simulink model "Model"  (R2020b)
settings: Solver=FixedStepDiscrete  StartTime=0.0  StopTime=inf  RelTol=1e-3
undefined symbols (not defined in the file): C12, designMultirateFIR, dt0
libraries: dspmlti4 x96, dspsrcs4 x89
(part 6 of 6)

== system Model/CORE_3_8/Path1/Mixer1 ==
  Input_I : Inport
  Input_Q : Inport  Port=2
  DDS_I : Inport  Port=3
  DDS_Q : Inport  Port=4
  Add : Sum
  Add1 : Sum
  Add2 : Sum  Inputs=-+
  Add3 : Sum  Inputs=+-
  Add4 : Sum
  Delay{1..11} (11 alike) : Delay  DelayLength=1  InitialCondition=0  SampleTime=dt0
  Product : Product
  Product1 : Product
  Product2 : Product
  Output_I : Outport
  Output_Q : Outport  Port=2
  wires:
  DDS_I/1 -> Delay9/1, Add/1
  Input_Q/1 -> Add2/2, Add1/2
  Add/1 -> Delay10/1
  Delay10/1 -> Product/2  "Sum1"
  Add2/1 -> Delay1/1
  Add1/1 -> Delay2/1
  Product/1 -> Delay3/1
  Delay3/1 -> Add4/1, Add3/1  "K1"
  Delay2/1 -> Product1/1  "Sum2"
  Product1/1 -> Delay4/1
  Delay4/1 -> Add3/2  "K2"
  Delay1/1 -> Product2/2  "Sum3"
  Product2/1 -> Delay5/1
  Delay5/1 -> Add4/2  "K3"
  Add3/1 -> Delay6/1
  Add4/1 -> Delay7/1
  Delay6/1 -> Output_I/1  "Sum4"
  Delay7/1 -> Output_Q/1  "Sum5"
  Input_I/1 -> Add2/1, Add1/1, Delay8/1
  DDS_Q/1 -> Delay11/1, Add/2
  Delay8/1 -> Product/1  "Input_I_w1"
  Delay11/1 -> Product1/2  "DDS_Q_w1"
  Delay9/1 -> Product2/1  "DDS_I_w1"

== system Model/CORE_3_8/Path2/DDS_Gen1 ==
  In1 : Inport
  Exp : Math  SaturateOnIntegerOverflow=on
  Gain : Gain  Gain=-1i*2*pi
  Product : Product
  Signal From Workspace1 : dspsrcs4/Signal From Workspace  X=t0  Ts=dt0  nsamps=1  OutputAfterFinalValue=Cyclic repetition  ignoreOrWarnInputAndFrameLengths=off  OutputFrames=off
  Out1 : Outport
  wires:
  Signal From Workspace1/1 -> Gain/1
  Exp/1 -> Out1/1
  Gain/1 -> Product/2
  Product/1 -> Exp/1
  In1/1 -> Product/1

== system Model/CORE_3_8/Path2/Mixer1 ==
  Input_I : Inport
  Input_Q : Inport  Port=2
  DDS_I : Inport  Port=3
  DDS_Q : Inport  Port=4
  Add : Sum
  Add1 : Sum
  Add2 : Sum  Inputs=-+
  Add3 : Sum  Inputs=+-
  Add4 : Sum
  Delay{1..11} (11 alike) : Delay  DelayLength=1  InitialCondition=0  SampleTime=dt0
  Product : Product
  Product1 : Product
  Product2 : Product
  Output_I : Outport
  Output_Q : Outport  Port=2
  wires:
  DDS_I/1 -> Delay9/1, Add/1
  Input_Q/1 -> Add2/2, Add1/2
  Add/1 -> Delay10/1
  Delay10/1 -> Product/2  "Sum1"
  Add2/1 -> Delay1/1
  Add1/1 -> Delay2/1
  Product/1 -> Delay3/1
  Delay3/1 -> Add4/1, Add3/1  "K1"
  Delay2/1 -> Product1/1  "Sum2"
  Product1/1 -> Delay4/1
  Delay4/1 -> Add3/2  "K2"
  Delay1/1 -> Product2/2  "Sum3"
  Product2/1 -> Delay5/1
  Delay5/1 -> Add4/2  "K3"
  Add3/1 -> Delay6/1
  Add4/1 -> Delay7/1
  Delay6/1 -> Output_I/1  "Sum4"
  Delay7/1 -> Output_Q/1  "Sum5"
  Input_I/1 -> Add2/1, Add1/1, Delay8/1
  DDS_Q/1 -> Delay11/1, Add/2
  Delay8/1 -> Product/1  "Input_I_w1"
  Delay11/1 -> Product1/2  "DDS_Q_w1"
  Delay9/1 -> Product2/1  "DDS_I_w1"

== system Model/CORE_3_8/Path3/DDS_Gen1 ==
  In1 : Inport
  Exp : Math  SaturateOnIntegerOverflow=on
  Gain : Gain  Gain=-1i*2*pi
  Product : Product
  Signal From Workspace1 : dspsrcs4/Signal From Workspace  X=t0  Ts=dt0  nsamps=1  OutputAfterFinalValue=Cyclic repetition  ignoreOrWarnInputAndFrameLengths=off  OutputFrames=off
  Out1 : Outport
  wires:
  Signal From Workspace1/1 -> Gain/1
  Exp/1 -> Out1/1
  Gain/1 -> Product/2
  Product/1 -> Exp/1
  In1/1 -> Product/1

== system Model/CORE_3_8/Path3/Mixer1 ==
  Input_I : Inport
  Input_Q : Inport  Port=2
  DDS_I : Inport  Port=3
  DDS_Q : Inport  Port=4
  Add : Sum
  Add1 : Sum
  Add2 : Sum  Inputs=-+
  Add3 : Sum  Inputs=+-
  Add4 : Sum
  Delay{1..11} (11 alike) : Delay  DelayLength=1  InitialCondition=0  SampleTime=dt0
  Product : Product
  Product1 : Product
  Product2 : Product
  Output_I : Outport
  Output_Q : Outport  Port=2
  wires:
  DDS_I/1 -> Delay9/1, Add/1
  Input_Q/1 -> Add2/2, Add1/2
  Add/1 -> Delay10/1
  Delay10/1 -> Product/2  "Sum1"
  Add2/1 -> Delay1/1
  Add1/1 -> Delay2/1
  Product/1 -> Delay3/1
  Delay3/1 -> Add4/1, Add3/1  "K1"
  Delay2/1 -> Product1/1  "Sum2"
  Product1/1 -> Delay4/1
  Delay4/1 -> Add3/2  "K2"
  Delay1/1 -> Product2/2  "Sum3"
  Product2/1 -> Delay5/1
  Delay5/1 -> Add4/2  "K3"
  Add3/1 -> Delay6/1
  Add4/1 -> Delay7/1
  Delay6/1 -> Output_I/1  "Sum4"
  Delay7/1 -> Output_Q/1  "Sum5"
  Input_I/1 -> Add2/1, Add1/1, Delay8/1
  DDS_Q/1 -> Delay11/1, Add/2
  Delay8/1 -> Product/1  "Input_I_w1"
  Delay11/1 -> Product1/2  "DDS_Q_w1"
  Delay9/1 -> Product2/1  "DDS_I_w1"

== system Model/CORE_3_8/Path4/DDS_Gen1 ==
  In1 : Inport
  Exp : Math  SaturateOnIntegerOverflow=on
  Gain : Gain  Gain=-1i*2*pi
  Product : Product
  Signal From Workspace1 : dspsrcs4/Signal From Workspace  X=t0  Ts=dt0  nsamps=1  OutputAfterFinalValue=Cyclic repetition  ignoreOrWarnInputAndFrameLengths=off  OutputFrames=off
  Out1 : Outport
  wires:
  Signal From Workspace1/1 -> Gain/1
  Exp/1 -> Out1/1
  Gain/1 -> Product/2
  Product/1 -> Exp/1
  In1/1 -> Product/1

== system Model/CORE_3_8/Path4/Mixer1 ==
  Input_I : Inport
  Input_Q : Inport  Port=2
  DDS_I : Inport  Port=3
  DDS_Q : Inport  Port=4
  Add : Sum
  Add1 : Sum
  Add2 : Sum  Inputs=-+
  Add3 : Sum  Inputs=+-
  Add4 : Sum
  Delay{1..11} (11 alike) : Delay  DelayLength=1  InitialCondition=0  SampleTime=dt0
  Product : Product
  Product1 : Product
  Product2 : Product
  Output_I : Outport
  Output_Q : Outport  Port=2
  wires:
  DDS_I/1 -> Delay9/1, Add/1
  Input_Q/1 -> Add2/2, Add1/2
  Add/1 -> Delay10/1
  Delay10/1 -> Product/2  "Sum1"
  Add2/1 -> Delay1/1
  Add1/1 -> Delay2/1
  Product/1 -> Delay3/1
  Delay3/1 -> Add4/1, Add3/1  "K1"
  Delay2/1 -> Product1/1  "Sum2"
  Product1/1 -> Delay4/1
  Delay4/1 -> Add3/2  "K2"
  Delay1/1 -> Product2/2  "Sum3"
  Product2/1 -> Delay5/1
  Delay5/1 -> Add4/2  "K3"
  Add3/1 -> Delay6/1
  Add4/1 -> Delay7/1
  Delay6/1 -> Output_I/1  "Sum4"
  Delay7/1 -> Output_Q/1  "Sum5"
  Input_I/1 -> Add2/1, Add1/1, Delay8/1
  DDS_Q/1 -> Delay11/1, Add/2
  Delay8/1 -> Product/1  "Input_I_w1"
  Delay11/1 -> Product1/2  "DDS_Q_w1"
  Delay9/1 -> Product2/1  "DDS_I_w1"

== system Model/CORE_3_8/Path5/DDS_Gen1 ==
  In1 : Inport
  Exp : Math  SaturateOnIntegerOverflow=on
  Gain : Gain  Gain=-1i*2*pi
  Product : Product
  Signal From Workspace1 : dspsrcs4/Signal From Workspace  X=t0  Ts=dt0  nsamps=1  OutputAfterFinalValue=Cyclic repetition  ignoreOrWarnInputAndFrameLengths=off  OutputFrames=off
  Out1 : Outport
  wires:
  Signal From Workspace1/1 -> Gain/1
  Exp/1 -> Out1/1
  Gain/1 -> Product/2
  Product/1 -> Exp/1
  In1/1 -> Product/1

== system Model/CORE_3_8/Path5/Mixer1 ==
  Input_I : Inport
  Input_Q : Inport  Port=2
  DDS_I : Inport  Port=3
  DDS_Q : Inport  Port=4
  Add : Sum
  Add1 : Sum
  Add2 : Sum  Inputs=-+
  Add3 : Sum  Inputs=+-
  Add4 : Sum
  Delay{1..11} (11 alike) : Delay  DelayLength=1  InitialCondition=0  SampleTime=dt0
  Product : Product
  Product1 : Product
  Product2 : Product
  Output_I : Outport
  Output_Q : Outport  Port=2
  wires:
  DDS_I/1 -> Delay9/1, Add/1
  Input_Q/1 -> Add2/2, Add1/2
  Add/1 -> Delay10/1
  Delay10/1 -> Product/2  "Sum1"
  Add2/1 -> Delay1/1
  Add1/1 -> Delay2/1
  Product/1 -> Delay3/1
  Delay3/1 -> Add4/1, Add3/1  "K1"
  Delay2/1 -> Product1/1  "Sum2"
  Product1/1 -> Delay4/1
  Delay4/1 -> Add3/2  "K2"
  Delay1/1 -> Product2/2  "Sum3"
  Product2/1 -> Delay5/1
  Delay5/1 -> Add4/2  "K3"
  Add3/1 -> Delay6/1
  Add4/1 -> Delay7/1
  Delay6/1 -> Output_I/1  "Sum4"
  Delay7/1 -> Output_Q/1  "Sum5"
  Input_I/1 -> Add2/1, Add1/1, Delay8/1
  DDS_Q/1 -> Delay11/1, Add/2
  Delay8/1 -> Product/1  "Input_I_w1"
  Delay11/1 -> Product1/2  "DDS_Q_w1"
  Delay9/1 -> Product2/1  "DDS_I_w1"

== system Model/CORE_3_8/Path6/DDS_Gen1 ==
  In1 : Inport
  Exp : Math  SaturateOnIntegerOverflow=on
  Gain : Gain  Gain=-1i*2*pi
  Product : Product
  Signal From Workspace1 : dspsrcs4/Signal From Workspace  X=t0  Ts=dt0  nsamps=1  OutputAfterFinalValue=Cyclic repetition  ignoreOrWarnInputAndFrameLengths=off  OutputFrames=off
  Out1 : Outport
  wires:
  Signal From Workspace1/1 -> Gain/1
  Exp/1 -> Out1/1
  Gain/1 -> Product/2
  Product/1 -> Exp/1
  In1/1 -> Product/1

== system Model/CORE_3_8/Path6/Mixer1 ==
  Input_I : Inport
  Input_Q : Inport  Port=2
  DDS_I : Inport  Port=3
  DDS_Q : Inport  Port=4
  Add : Sum
  Add1 : Sum
  Add2 : Sum  Inputs=-+
  Add3 : Sum  Inputs=+-
  Add4 : Sum
  Delay{1..11} (11 alike) : Delay  DelayLength=1  InitialCondition=0  SampleTime=dt0
  Product : Product
  Product1 : Product
  Product2 : Product
  Output_I : Outport
  Output_Q : Outport  Port=2
  wires:
  DDS_I/1 -> Delay9/1, Add/1
  Input_Q/1 -> Add2/2, Add1/2
  Add/1 -> Delay10/1
  Delay10/1 -> Product/2  "Sum1"
  Add2/1 -> Delay1/1
  Add1/1 -> Delay2/1
  Product/1 -> Delay3/1
  Delay3/1 -> Add4/1, Add3/1  "K1"
  Delay2/1 -> Product1/1  "Sum2"
  Product1/1 -> Delay4/1
  Delay4/1 -> Add3/2  "K2"
  Delay1/1 -> Product2/2  "Sum3"
  Product2/1 -> Delay5/1
  Delay5/1 -> Add4/2  "K3"
  Add3/1 -> Delay6/1
  Add4/1 -> Delay7/1
  Delay6/1 -> Output_I/1  "Sum4"
  Delay7/1 -> Output_Q/1  "Sum5"
  Input_I/1 -> Add2/1, Add1/1, Delay8/1
  DDS_Q/1 -> Delay11/1, Add/2
  Delay8/1 -> Product/1  "Input_I_w1"
  Delay11/1 -> Product1/2  "DDS_Q_w1"
  Delay9/1 -> Product2/1  "DDS_I_w1"

== system Model/CORE_3_8/Path7/DDS_Gen1 ==
  In1 : Inport
  Exp : Math  SaturateOnIntegerOverflow=on
  Gain : Gain  Gain=-1i*2*pi
  Product : Product
  Signal From Workspace1 : dspsrcs4/Signal From Workspace  X=t0  Ts=dt0  nsamps=1  OutputAfterFinalValue=Cyclic repetition  ignoreOrWarnInputAndFrameLengths=off  OutputFrames=off
  Out1 : Outport
  wires:
  Signal From Workspace1/1 -> Gain/1
  Exp/1 -> Out1/1
  Gain/1 -> Product/2
  Product/1 -> Exp/1
  In1/1 -> Product/1

== system Model/CORE_3_8/Path7/Mixer1 ==
  Input_I : Inport
  Input_Q : Inport  Port=2
  DDS_I : Inport  Port=3
  DDS_Q : Inport  Port=4
  Add : Sum
  Add1 : Sum
  Add2 : Sum  Inputs=-+
  Add3 : Sum  Inputs=+-
  Add4 : Sum
  Delay{1..11} (11 alike) : Delay  DelayLength=1  InitialCondition=0  SampleTime=dt0
  Product : Product
  Product1 : Product
  Product2 : Product
  Output_I : Outport
  Output_Q : Outport  Port=2
  wires:
  DDS_I/1 -> Delay9/1, Add/1
  Input_Q/1 -> Add2/2, Add1/2
  Add/1 -> Delay10/1
  Delay10/1 -> Product/2  "Sum1"
  Add2/1 -> Delay1/1
  Add1/1 -> Delay2/1
  Product/1 -> Delay3/1
  Delay3/1 -> Add4/1, Add3/1  "K1"
  Delay2/1 -> Product1/1  "Sum2"
  Product1/1 -> Delay4/1
  Delay4/1 -> Add3/2  "K2"
  Delay1/1 -> Product2/2  "Sum3"
  Product2/1 -> Delay5/1
  Delay5/1 -> Add4/2  "K3"
  Add3/1 -> Delay6/1
  Add4/1 -> Delay7/1
  Delay6/1 -> Output_I/1  "Sum4"
  Delay7/1 -> Output_Q/1  "Sum5"
  Input_I/1 -> Add2/1, Add1/1, Delay8/1
  DDS_Q/1 -> Delay11/1, Add/2
  Delay8/1 -> Product/1  "Input_I_w1"
  Delay11/1 -> Product1/2  "DDS_Q_w1"
  Delay9/1 -> Product2/1  "DDS_I_w1"

== system Model/CORE_3_8/Path8/DDS_Gen1 ==
  In1 : Inport
  Exp : Math  SaturateOnIntegerOverflow=on
  Gain : Gain  Gain=-1i*2*pi
  Product : Product
  Signal From Workspace1 : dspsrcs4/Signal From Workspace  X=t0  Ts=dt0  nsamps=1  OutputAfterFinalValue=Cyclic repetition  ignoreOrWarnInputAndFrameLengths=off  OutputFrames=off
  Out1 : Outport
  wires:
  Signal From Workspace1/1 -> Gain/1
  Exp/1 -> Out1/1
  Gain/1 -> Product/2
  Product/1 -> Exp/1
  In1/1 -> Product/1

== system Model/CORE_3_8/Path8/Mixer1 ==
  Input_I : Inport
  Input_Q : Inport  Port=2
  DDS_I : Inport  Port=3
  DDS_Q : Inport  Port=4
  Add : Sum
  Add1 : Sum
  Add2 : Sum  Inputs=-+
  Add3 : Sum  Inputs=+-
  Add4 : Sum
  Delay{1..11} (11 alike) : Delay  DelayLength=1  InitialCondition=0  SampleTime=dt0
  Product : Product
  Product1 : Product
  Product2 : Product
  Output_I : Outport
  Output_Q : Outport  Port=2
  wires:
  DDS_I/1 -> Delay9/1, Add/1
  Input_Q/1 -> Add2/2, Add1/2
  Add/1 -> Delay10/1
  Delay10/1 -> Product/2  "Sum1"
  Add2/1 -> Delay1/1
  Add1/1 -> Delay2/1
  Product/1 -> Delay3/1
  Delay3/1 -> Add4/1, Add3/1  "K1"
  Delay2/1 -> Product1/1  "Sum2"
  Product1/1 -> Delay4/1
  Delay4/1 -> Add3/2  "K2"
  Delay1/1 -> Product2/2  "Sum3"
  Product2/1 -> Delay5/1
  Delay5/1 -> Add4/2  "K3"
  Add3/1 -> Delay6/1
  Add4/1 -> Delay7/1
  Delay6/1 -> Output_I/1  "Sum4"
  Delay7/1 -> Output_Q/1  "Sum5"
  Input_I/1 -> Add2/1, Add1/1, Delay8/1
  DDS_Q/1 -> Delay11/1, Add/2
  Delay8/1 -> Product/1  "Input_I_w1"
  Delay11/1 -> Product1/2  "DDS_Q_w1"
  Delay9/1 -> Product2/1  "DDS_I_w1"

== system Model/CORE_3_9/Path1/DDS_Gen1 ==
  In1 : Inport
  Exp : Math  SaturateOnIntegerOverflow=on
  Gain : Gain  Gain=-1i*2*pi
  Product : Product
  Signal From Workspace1 : dspsrcs4/Signal From Workspace  X=t0  Ts=dt0  nsamps=1  OutputAfterFinalValue=Cyclic repetition  ignoreOrWarnInputAndFrameLengths=off  OutputFrames=off
  Out1 : Outport
  wires:
  Signal From Workspace1/1 -> Gain/1
  Exp/1 -> Out1/1
  Gain/1 -> Product/2
  Product/1 -> Exp/1
  In1/1 -> Product/1

== system Model/CORE_3_9/Path1/Mixer1 ==
  Input_I : Inport
  Input_Q : Inport  Port=2
  DDS_I : Inport  Port=3
  DDS_Q : Inport  Port=4
  Add : Sum
  Add1 : Sum
  Add2 : Sum  Inputs=-+
  Add3 : Sum  Inputs=+-
  Add4 : Sum
  Delay{1..11} (11 alike) : Delay  DelayLength=1  InitialCondition=0  SampleTime=dt0
  Product : Product
  Product1 : Product
  Product2 : Product
  Output_I : Outport
  Output_Q : Outport  Port=2
  wires:
  DDS_I/1 -> Delay9/1, Add/1
  Input_Q/1 -> Add2/2, Add1/2
  Add/1 -> Delay10/1
  Delay10/1 -> Product/2  "Sum1"
  Add2/1 -> Delay1/1
  Add1/1 -> Delay2/1
  Product/1 -> Delay3/1
  Delay3/1 -> Add4/1, Add3/1  "K1"
  Delay2/1 -> Product1/1  "Sum2"
  Product1/1 -> Delay4/1
  Delay4/1 -> Add3/2  "K2"
  Delay1/1 -> Product2/2  "Sum3"
  Product2/1 -> Delay5/1
  Delay5/1 -> Add4/2  "K3"
  Add3/1 -> Delay6/1
  Add4/1 -> Delay7/1
  Delay6/1 -> Output_I/1  "Sum4"
  Delay7/1 -> Output_Q/1  "Sum5"
  Input_I/1 -> Add2/1, Add1/1, Delay8/1
  DDS_Q/1 -> Delay11/1, Add/2
  Delay8/1 -> Product/1  "Input_I_w1"
  Delay11/1 -> Product1/2  "DDS_Q_w1"
  Delay9/1 -> Product2/1  "DDS_I_w1"

== system Model/CORE_3_9/Path2/DDS_Gen1 ==
  In1 : Inport
  Exp : Math  SaturateOnIntegerOverflow=on
  Gain : Gain  Gain=-1i*2*pi
  Product : Product
  Signal From Workspace1 : dspsrcs4/Signal From Workspace  X=t0  Ts=dt0  nsamps=1  OutputAfterFinalValue=Cyclic repetition  ignoreOrWarnInputAndFrameLengths=off  OutputFrames=off
  Out1 : Outport
  wires:
  Signal From Workspace1/1 -> Gain/1
  Exp/1 -> Out1/1
  Gain/1 -> Product/2
  Product/1 -> Exp/1
  In1/1 -> Product/1

== system Model/CORE_3_9/Path2/Mixer1 ==
  Input_I : Inport
  Input_Q : Inport  Port=2
  DDS_I : Inport  Port=3
  DDS_Q : Inport  Port=4
  Add : Sum
  Add1 : Sum
  Add2 : Sum  Inputs=-+
  Add3 : Sum  Inputs=+-
  Add4 : Sum
  Delay{1..11} (11 alike) : Delay  DelayLength=1  InitialCondition=0  SampleTime=dt0
  Product : Product
  Product1 : Product
  Product2 : Product
  Output_I : Outport
  Output_Q : Outport  Port=2
  wires:
  DDS_I/1 -> Delay9/1, Add/1
  Input_Q/1 -> Add2/2, Add1/2
  Add/1 -> Delay10/1
  Delay10/1 -> Product/2  "Sum1"
  Add2/1 -> Delay1/1
  Add1/1 -> Delay2/1
  Product/1 -> Delay3/1
  Delay3/1 -> Add4/1, Add3/1  "K1"
  Delay2/1 -> Product1/1  "Sum2"
  Product1/1 -> Delay4/1
  Delay4/1 -> Add3/2  "K2"
  Delay1/1 -> Product2/2  "Sum3"
  Product2/1 -> Delay5/1
  Delay5/1 -> Add4/2  "K3"
  Add3/1 -> Delay6/1
  Add4/1 -> Delay7/1
  Delay6/1 -> Output_I/1  "Sum4"
  Delay7/1 -> Output_Q/1  "Sum5"
  Input_I/1 -> Add2/1, Add1/1, Delay8/1
  DDS_Q/1 -> Delay11/1, Add/2
  Delay8/1 -> Product/1  "Input_I_w1"
  Delay11/1 -> Product1/2  "DDS_Q_w1"
  Delay9/1 -> Product2/1  "DDS_I_w1"

== system Model/CORE_3_9/Path3/DDS_Gen1 ==
  In1 : Inport
  Exp : Math  SaturateOnIntegerOverflow=on
  Gain : Gain  Gain=-1i*2*pi
  Product : Product
  Signal From Workspace1 : dspsrcs4/Signal From Workspace  X=t0  Ts=dt0  nsamps=1  OutputAfterFinalValue=Cyclic repetition  ignoreOrWarnInputAndFrameLengths=off  OutputFrames=off
  Out1 : Outport
  wires:
  Signal From Workspace1/1 -> Gain/1
  Exp/1 -> Out1/1
  Gain/1 -> Product/2
  Product/1 -> Exp/1
  In1/1 -> Product/1

== system Model/CORE_3_9/Path3/Mixer1 ==
  Input_I : Inport
  Input_Q : Inport  Port=2
  DDS_I : Inport  Port=3
  DDS_Q : Inport  Port=4
  Add : Sum
  Add1 : Sum
  Add2 : Sum  Inputs=-+
  Add3 : Sum  Inputs=+-
  Add4 : Sum
  Delay{1..11} (11 alike) : Delay  DelayLength=1  InitialCondition=0  SampleTime=dt0
  Product : Product
  Product1 : Product
  Product2 : Product
  Output_I : Outport
  Output_Q : Outport  Port=2
  wires:
  DDS_I/1 -> Delay9/1, Add/1
  Input_Q/1 -> Add2/2, Add1/2
  Add/1 -> Delay10/1
  Delay10/1 -> Product/2  "Sum1"
  Add2/1 -> Delay1/1
  Add1/1 -> Delay2/1
  Product/1 -> Delay3/1
  Delay3/1 -> Add4/1, Add3/1  "K1"
  Delay2/1 -> Product1/1  "Sum2"
  Product1/1 -> Delay4/1
  Delay4/1 -> Add3/2  "K2"
  Delay1/1 -> Product2/2  "Sum3"
  Product2/1 -> Delay5/1
  Delay5/1 -> Add4/2  "K3"
  Add3/1 -> Delay6/1
  Add4/1 -> Delay7/1
  Delay6/1 -> Output_I/1  "Sum4"
  Delay7/1 -> Output_Q/1  "Sum5"
  Input_I/1 -> Add2/1, Add1/1, Delay8/1
  DDS_Q/1 -> Delay11/1, Add/2
  Delay8/1 -> Product/1  "Input_I_w1"
  Delay11/1 -> Product1/2  "DDS_Q_w1"
  Delay9/1 -> Product2/1  "DDS_I_w1"

== system Model/CORE_3_9/Path4/DDS_Gen1 ==
  In1 : Inport
  Exp : Math  SaturateOnIntegerOverflow=on
  Gain : Gain  Gain=-1i*2*pi
  Product : Product
  Signal From Workspace1 : dspsrcs4/Signal From Workspace  X=t0  Ts=dt0  nsamps=1  OutputAfterFinalValue=Cyclic repetition  ignoreOrWarnInputAndFrameLengths=off  OutputFrames=off
  Out1 : Outport
  wires:
  Signal From Workspace1/1 -> Gain/1
  Exp/1 -> Out1/1
  Gain/1 -> Product/2
  Product/1 -> Exp/1
  In1/1 -> Product/1

== system Model/CORE_3_9/Path4/Mixer1 ==
  Input_I : Inport
  Input_Q : Inport  Port=2
  DDS_I : Inport  Port=3
  DDS_Q : Inport  Port=4
  Add : Sum
  Add1 : Sum
  Add2 : Sum  Inputs=-+
  Add3 : Sum  Inputs=+-
  Add4 : Sum
  Delay{1..11} (11 alike) : Delay  DelayLength=1  InitialCondition=0  SampleTime=dt0
  Product : Product
  Product1 : Product
  Product2 : Product
  Output_I : Outport
  Output_Q : Outport  Port=2
  wires:
  DDS_I/1 -> Delay9/1, Add/1
  Input_Q/1 -> Add2/2, Add1/2
  Add/1 -> Delay10/1
  Delay10/1 -> Product/2  "Sum1"
  Add2/1 -> Delay1/1
  Add1/1 -> Delay2/1
  Product/1 -> Delay3/1
  Delay3/1 -> Add4/1, Add3/1  "K1"
  Delay2/1 -> Product1/1  "Sum2"
  Product1/1 -> Delay4/1
  Delay4/1 -> Add3/2  "K2"
  Delay1/1 -> Product2/2  "Sum3"
  Product2/1 -> Delay5/1
  Delay5/1 -> Add4/2  "K3"
  Add3/1 -> Delay6/1
  Add4/1 -> Delay7/1
  Delay6/1 -> Output_I/1  "Sum4"
  Delay7/1 -> Output_Q/1  "Sum5"
  Input_I/1 -> Add2/1, Add1/1, Delay8/1
  DDS_Q/1 -> Delay11/1, Add/2
  Delay8/1 -> Product/1  "Input_I_w1"
  Delay11/1 -> Product1/2  "DDS_Q_w1"
  Delay9/1 -> Product2/1  "DDS_I_w1"

== system Model/CORE_3_9/Path5/DDS_Gen1 ==
  In1 : Inport
  Exp : Math  SaturateOnIntegerOverflow=on
  Gain : Gain  Gain=-1i*2*pi
  Product : Product
  Signal From Workspace1 : dspsrcs4/Signal From Workspace  X=t0  Ts=dt0  nsamps=1  OutputAfterFinalValue=Cyclic repetition  ignoreOrWarnInputAndFrameLengths=off  OutputFrames=off
  Out1 : Outport
  wires:
  Signal From Workspace1/1 -> Gain/1
  Exp/1 -> Out1/1
  Gain/1 -> Product/2
  Product/1 -> Exp/1
  In1/1 -> Product/1

== system Model/CORE_3_9/Path5/Mixer1 ==
  Input_I : Inport
  Input_Q : Inport  Port=2
  DDS_I : Inport  Port=3
  DDS_Q : Inport  Port=4
  Add : Sum
  Add1 : Sum
  Add2 : Sum  Inputs=-+
  Add3 : Sum  Inputs=+-
  Add4 : Sum
  Delay{1..11} (11 alike) : Delay  DelayLength=1  InitialCondition=0  SampleTime=dt0
  Product : Product
  Product1 : Product
  Product2 : Product
  Output_I : Outport
  Output_Q : Outport  Port=2
  wires:
  DDS_I/1 -> Delay9/1, Add/1
  Input_Q/1 -> Add2/2, Add1/2
  Add/1 -> Delay10/1
  Delay10/1 -> Product/2  "Sum1"
  Add2/1 -> Delay1/1
  Add1/1 -> Delay2/1
  Product/1 -> Delay3/1
  Delay3/1 -> Add4/1, Add3/1  "K1"
  Delay2/1 -> Product1/1  "Sum2"
  Product1/1 -> Delay4/1
  Delay4/1 -> Add3/2  "K2"
  Delay1/1 -> Product2/2  "Sum3"
  Product2/1 -> Delay5/1
  Delay5/1 -> Add4/2  "K3"
  Add3/1 -> Delay6/1
  Add4/1 -> Delay7/1
  Delay6/1 -> Output_I/1  "Sum4"
  Delay7/1 -> Output_Q/1  "Sum5"
  Input_I/1 -> Add2/1, Add1/1, Delay8/1
  DDS_Q/1 -> Delay11/1, Add/2
  Delay8/1 -> Product/1  "Input_I_w1"
  Delay11/1 -> Product1/2  "DDS_Q_w1"
  Delay9/1 -> Product2/1  "DDS_I_w1"

== system Model/CORE_3_9/Path6/DDS_Gen1 ==
  In1 : Inport
  Exp : Math  SaturateOnIntegerOverflow=on
  Gain : Gain  Gain=-1i*2*pi
  Product : Product
  Signal From Workspace1 : dspsrcs4/Signal From Workspace  X=t0  Ts=dt0  nsamps=1  OutputAfterFinalValue=Cyclic repetition  ignoreOrWarnInputAndFrameLengths=off  OutputFrames=off
  Out1 : Outport
  wires:
  Signal From Workspace1/1 -> Gain/1
  Exp/1 -> Out1/1
  Gain/1 -> Product/2
  Product/1 -> Exp/1
  In1/1 -> Product/1

== system Model/CORE_3_9/Path6/Mixer1 ==
  Input_I : Inport
  Input_Q : Inport  Port=2
  DDS_I : Inport  Port=3
  DDS_Q : Inport  Port=4
  Add : Sum
  Add1 : Sum
  Add2 : Sum  Inputs=-+
  Add3 : Sum  Inputs=+-
  Add4 : Sum
  Delay{1..11} (11 alike) : Delay  DelayLength=1  InitialCondition=0  SampleTime=dt0
  Product : Product
  Product1 : Product
  Product2 : Product
  Output_I : Outport
  Output_Q : Outport  Port=2
  wires:
  DDS_I/1 -> Delay9/1, Add/1
  Input_Q/1 -> Add2/2, Add1/2
  Add/1 -> Delay10/1
  Delay10/1 -> Product/2  "Sum1"
  Add2/1 -> Delay1/1
  Add1/1 -> Delay2/1
  Product/1 -> Delay3/1
  Delay3/1 -> Add4/1, Add3/1  "K1"
  Delay2/1 -> Product1/1  "Sum2"
  Product1/1 -> Delay4/1
  Delay4/1 -> Add3/2  "K2"
  Delay1/1 -> Product2/2  "Sum3"
  Product2/1 -> Delay5/1
  Delay5/1 -> Add4/2  "K3"
  Add3/1 -> Delay6/1
  Add4/1 -> Delay7/1
  Delay6/1 -> Output_I/1  "Sum4"
  Delay7/1 -> Output_Q/1  "Sum5"
  Input_I/1 -> Add2/1, Add1/1, Delay8/1
  DDS_Q/1 -> Delay11/1, Add/2
  Delay8/1 -> Product/1  "Input_I_w1"
  Delay11/1 -> Product1/2  "DDS_Q_w1"
  Delay9/1 -> Product2/1  "DDS_I_w1"

== system Model/CORE_3_9/Path7/DDS_Gen1 ==
  In1 : Inport
  Exp : Math  SaturateOnIntegerOverflow=on
  Gain : Gain  Gain=-1i*2*pi
  Product : Product
  Signal From Workspace1 : dspsrcs4/Signal From Workspace  X=t0  Ts=dt0  nsamps=1  OutputAfterFinalValue=Cyclic repetition  ignoreOrWarnInputAndFrameLengths=off  OutputFrames=off
  Out1 : Outport
  wires:
  Signal From Workspace1/1 -> Gain/1
  Exp/1 -> Out1/1
  Gain/1 -> Product/2
  Product/1 -> Exp/1
  In1/1 -> Product/1

== system Model/CORE_3_9/Path7/Mixer1 ==
  Input_I : Inport
  Input_Q : Inport  Port=2
  DDS_I : Inport  Port=3
  DDS_Q : Inport  Port=4
  Add : Sum
  Add1 : Sum
  Add2 : Sum  Inputs=-+
  Add3 : Sum  Inputs=+-
  Add4 : Sum
  Delay{1..11} (11 alike) : Delay  DelayLength=1  InitialCondition=0  SampleTime=dt0
  Product : Product
  Product1 : Product
  Product2 : Product
  Output_I : Outport
  Output_Q : Outport  Port=2
  wires:
  DDS_I/1 -> Delay9/1, Add/1
  Input_Q/1 -> Add2/2, Add1/2
  Add/1 -> Delay10/1
  Delay10/1 -> Product/2  "Sum1"
  Add2/1 -> Delay1/1
  Add1/1 -> Delay2/1
  Product/1 -> Delay3/1
  Delay3/1 -> Add4/1, Add3/1  "K1"
  Delay2/1 -> Product1/1  "Sum2"
  Product1/1 -> Delay4/1
  Delay4/1 -> Add3/2  "K2"
  Delay1/1 -> Product2/2  "Sum3"
  Product2/1 -> Delay5/1
  Delay5/1 -> Add4/2  "K3"
  Add3/1 -> Delay6/1
  Add4/1 -> Delay7/1
  Delay6/1 -> Output_I/1  "Sum4"
  Delay7/1 -> Output_Q/1  "Sum5"
  Input_I/1 -> Add2/1, Add1/1, Delay8/1
  DDS_Q/1 -> Delay11/1, Add/2
  Delay8/1 -> Product/1  "Input_I_w1"
  Delay11/1 -> Product1/2  "DDS_Q_w1"
  Delay9/1 -> Product2/1  "DDS_I_w1"

== system Model/CORE_3_9/Path8/DDS_Gen1 ==
  In1 : Inport
  Exp : Math  SaturateOnIntegerOverflow=on
  Gain : Gain  Gain=-1i*2*pi
  Product : Product
  Signal From Workspace1 : dspsrcs4/Signal From Workspace  X=t0  Ts=dt0  nsamps=1  OutputAfterFinalValue=Cyclic repetition  ignoreOrWarnInputAndFrameLengths=off  OutputFrames=off
  Out1 : Outport
  wires:
  Signal From Workspace1/1 -> Gain/1
  Exp/1 -> Out1/1
  Gain/1 -> Product/2
  Product/1 -> Exp/1
  In1/1 -> Product/1

== system Model/CORE_3_9/Path8/Mixer1 ==
  Input_I : Inport
  Input_Q : Inport  Port=2
  DDS_I : Inport  Port=3
  DDS_Q : Inport  Port=4
  Add : Sum
  Add1 : Sum
  Add2 : Sum  Inputs=-+
  Add3 : Sum  Inputs=+-
  Add4 : Sum
  Delay{1..11} (11 alike) : Delay  DelayLength=1  InitialCondition=0  SampleTime=dt0
  Product : Product
  Product1 : Product
  Product2 : Product
  Output_I : Outport
  Output_Q : Outport  Port=2
  wires:
  DDS_I/1 -> Delay9/1, Add/1
  Input_Q/1 -> Add2/2, Add1/2
  Add/1 -> Delay10/1
  Delay10/1 -> Product/2  "Sum1"
  Add2/1 -> Delay1/1
  Add1/1 -> Delay2/1
  Product/1 -> Delay3/1
  Delay3/1 -> Add4/1, Add3/1  "K1"
  Delay2/1 -> Product1/1  "Sum2"
  Product1/1 -> Delay4/1
  Delay4/1 -> Add3/2  "K2"
  Delay1/1 -> Product2/2  "Sum3"
  Product2/1 -> Delay5/1
  Delay5/1 -> Add4/2  "K3"
  Add3/1 -> Delay6/1
  Add4/1 -> Delay7/1
  Delay6/1 -> Output_I/1  "Sum4"
  Delay7/1 -> Output_Q/1  "Sum5"
  Input_I/1 -> Add2/1, Add1/1, Delay8/1
  DDS_Q/1 -> Delay11/1, Add/2
  Delay8/1 -> Product/1  "Input_I_w1"
  Delay11/1 -> Product1/2  "DDS_Q_w1"
  Delay9/1 -> Product2/1  "DDS_I_w1"
